simulink model "opdracht3"  (Simulink 6.6)
settings: Solver=ode45  StartTime=0.0  StopTime=inf  RelTol=1e-3
libraries: simulink x3, dspsrcs4 x1, simulink_extras x1
settings Model: Creator=student  LastModifiedBy=student

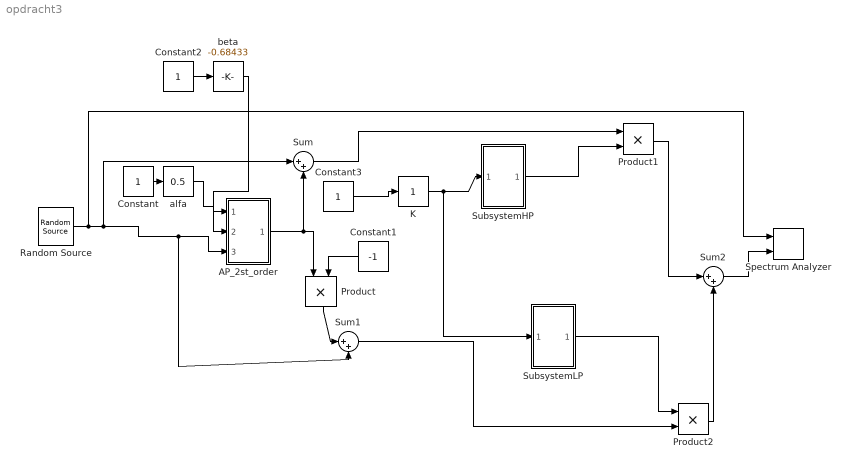
== system opdracht3 ==
  AP_2st_order : Subsystem
  Constant : Constant
  Constant1 : Constant  Orientation=left  Value=-1
  Constant2 : Constant
  Constant3 : Constant
  K : simulink/Math Operations/Slider Gain  SystemSampleTime=-1  low=0  gain=1  high=1
  Product : Product  Orientation=down  RndMeth=Zero
  Product1 : Product  RndMeth=Zero
  Product2 : Product  RndMeth=Zero
  Random Source : dspsrcs4/Random Source  SrcType=Uniform  NormMethod=Ziggurat  CltLength=12  MinVal=-10  MaxVal=10  MeanVal=0  VarVal=1  RepMode=Not repeatable  rawSeed=1  IsInherit=off  SampMode=Discrete  SampTime=1  SampFrame=1  DataType=Double  OutComplex=Real
  Spectrum Analyzer : simulink_extras/Additional Sinks/Spectrum Analyzer  SystemSampleTime=-1  npts=1024  fftpts=1024  HowOften=64  sampleT=1
  SubsystemHP : Subsystem
  SubsystemLP : Subsystem
  Sum : Sum  Inputs=|++
  Sum1 : Sum  Inputs=|++
  Sum2 : Sum  Inputs=|++
  alfa : simulink/Math Operations/Slider Gain  SystemSampleTime=-1  low=0  gain=0.5  high=1
  beta : simulink/Math Operations/Slider Gain  SystemSampleTime=-1  low=-0.9  gain=-0.68433  high=0.9
  wires:
  alfa/1 -> AP_2st_order/2(alfa)
  Constant/1 -> alfa/1
  Constant1/1 -> Product/2
  Product/1 -> Sum1/1
  Random Source/1 -> Sum1/2, AP_2st_order/3(source), Sum/1, Spectrum Analyzer/1
  Product1/1 -> Sum2/1
  Product2/1 -> Sum2/2
  Sum2/1 -> Spectrum Analyzer/2
  Sum/1 -> Product1/1
  Constant3/1 -> K/1
  K/1 -> SubsystemLP/1(In1), SubsystemHP/1(In1)
  SubsystemHP/1(Out1) -> Product1/2
  Sum1/1 -> Product2/2
  SubsystemLP/1(Out1) -> Product2/1
  AP_2st_order/1(Out1) -> Product/1, Sum/2
  Constant2/1 -> beta/1
  beta/1 -> AP_2st_order/1(beta)

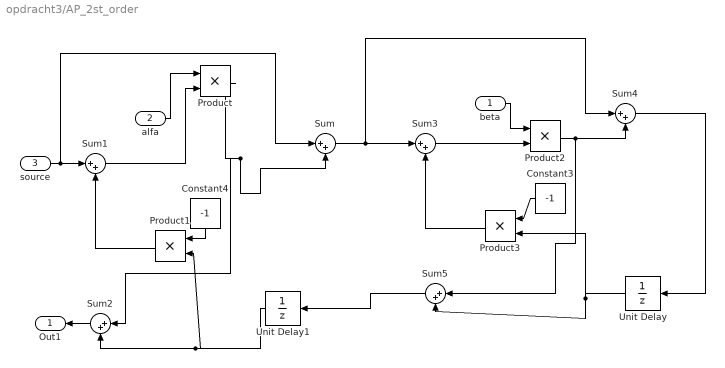
== system opdracht3/AP_2st_order ==
  beta : Inport
  alfa : Inport  Port=2
  source : Inport  Port=3
  Constant3 : Constant  Orientation=left  Value=-1
  Constant4 : Constant  Orientation=down  Value=-1
  Product : Product  RndMeth=Zero
  Product1 : Product  Orientation=left  RndMeth=Zero
  Product2 : Product  RndMeth=Zero
  Product3 : Product  Orientation=left  RndMeth=Zero
  Sum{,1,3..4} (4 alike) : Sum  Inputs=|++
  Sum2 : Sum  Orientation=left  Inputs=|++
  Sum5 : Sum  Orientation=left  Inputs=|++
  Unit Delay : UnitDelay  Orientation=left
  Unit Delay1 : UnitDelay  Orientation=left
  Out1 : Outport  Orientation=left
  wires:
  Sum1/1 -> Product/2
  Product1/1 -> Sum1/2
  Product/1 -> Sum/2, Sum2/1
  Sum/1 -> Sum3/1, Sum4/1
  Sum3/1 -> Product2/2
  Product2/1 -> Sum4/2, Sum5/1
  Sum4/1 -> Unit Delay/1
  Unit Delay/1 -> Sum5/2, Product3/2
  Product3/1 -> Sum3/2
  Constant3/1 -> Product3/1
  Sum5/1 -> Unit Delay1/1
  Unit Delay1/1 -> Sum2/2, Product1/2
  Constant4/1 -> Product1/1
  source/1 -> Sum1/1, Sum/1
  beta/1 -> Product2/1
  alfa/1 -> Product/1
  Sum2/1 -> Out1/1

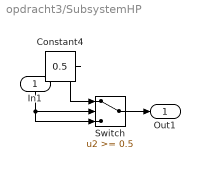
== system opdracht3/SubsystemHP ==
  In1 : Inport  Orientation=down
  Constant4 : Constant  Value=0.5
  Switch : Switch  Threshold=0.5
  Out1 : Outport
  wires:
  Constant4/1 -> Switch/1
  In1/1 -> Switch/3, Switch/2
  Switch/1 -> Out1/1

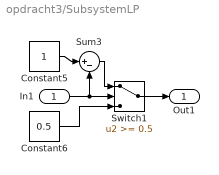
== system opdracht3/SubsystemLP ==
  In1 : Inport
  Constant5 : Constant
  Constant6 : Constant  Value=0.5
  Sum3 : Sum  Inputs=|+-
  Switch1 : Switch  Threshold=0.5
  Out1 : Outport
  wires:
  Sum3/1 -> Switch1/1
  Constant5/1 -> Sum3/1
  Constant6/1 -> Switch1/3
  In1/1 -> Switch1/2, Sum3/2
  Switch1/1 -> Out1/1
